simulink library "se_batching"  (Simulink 7.9)
settings: Solver=VariableStepDiscrete  SolverMode=SingleTasking  StartTime=0.0  StopTime=inf  RelTol=1e-3
libraries: simulink x7
settings Model: Creator=rrosson  LastModifiedBy=tsprock3

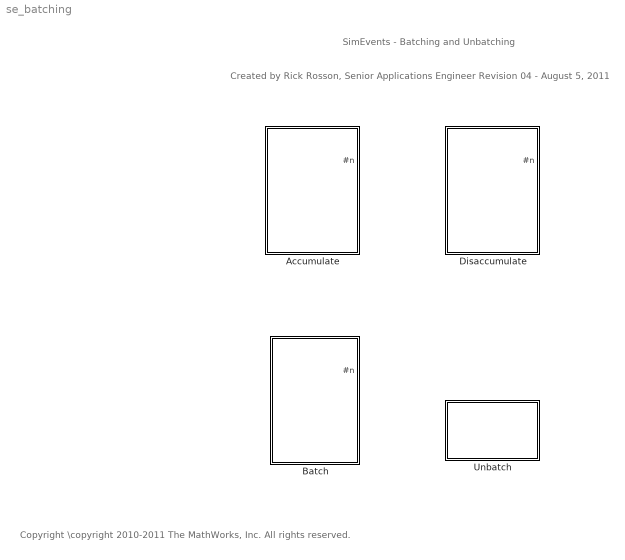
== system se_batching ==
  note: Copyright \copyright 2010-2011 The MathWorks, Inc. All rights reserved.
  note: SimEvents - Batching and Unbatching
  note: Created by Rick Rosson, Senior Applications Engineer
      | Revision 04 - August 5, 2011
  Accumulate : Subsystem  mask(Accumulate){Q=20}
      mask prompts: Q "Bach quantity (entities/batch), Q ="
      mask help:
      | Takes in entities and stores them until the number of entities stored reaches a specified number called the batch quantity.  The block then passes all of the stored entities to the output simultaneously.
      | The #n output signal provides the number of entities stored in the block at each time step.
      mask init:
      | if Q < 2
      |     error('Q must be greater than 1');
      | end
  Batch : Subsystem  mask(Batch){Q=20}
      mask prompts: Q "Bach quantity (entities/batch), Q ="
      mask help:
      | Takes in entities and stores them until the number of entities stored reaches a specified number called the batch quantity.  The block then generates a single entity, which represents a batch, and passes the batch entity to the output.
      | The #n output signal provides the number of entities stored in the block at each time step.
      mask init:
      | if Q < 2
      |     error('Q must be greater than 1');
      | end
  Disaccumulate : Subsystem  mask(Disaccumulaton){Qmax=inf, Nmax=inf, Tc=1}
      mask prompts: Qmax "Maxiumum batch size (entities per batch), Qmax"; Nmax "Maximum number of batches, Nmax ="; Tc "Cycle time, Tc ="
  Unbatch : Subsystem  mask(Unbatch){Q=20}
      mask prompts: Q "Batch quantity (entities/batch), Q ="
      mask help: Takes a single entity representing a batch and converts it into multiple entities. A parameter determines the batch quantity, which is the number of entities generated at the output for each entity arriving at the input.
      mask init:
      | if Q < 2
      |     error('Q must be greater than 1');
      | end

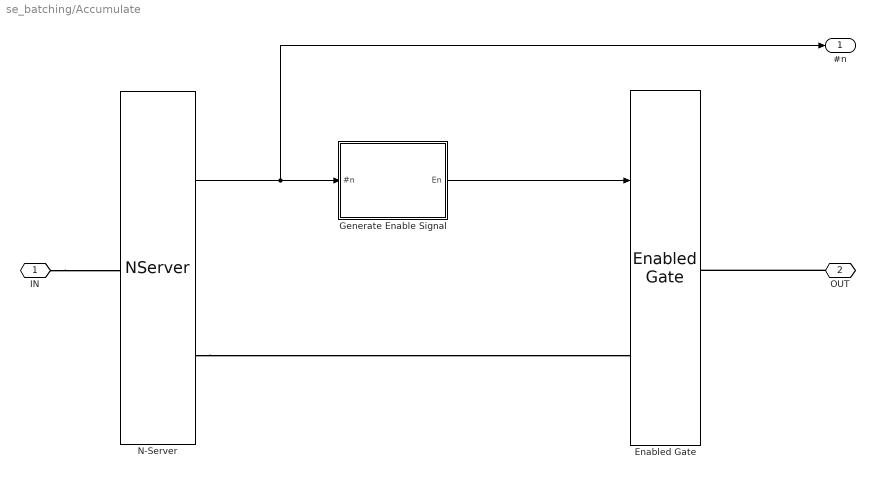
== system se_batching/Accumulate ==
  Enabled Gate : EnabledGate
  Generate Enable Signal : Subsystem
  N-Server : NServer  NumberOfServers=Q  ServiceTime=0  StatNumberInBlock=on
      settings: OutputPortMap=o1
  IN : PMIOPort  Port=1  Side=Left
  OUT : PMIOPort  Port=2  Side=Right
  #n : Outport
  wires:
  Generate Enable Signal/1(En) -> Enabled Gate/1
  N-Server/1 -> #n/1, Generate Enable Signal/1(#n)
  connections:
  OUT/RConn1 -- Enabled Gate/RConn1
  IN/RConn1 -- N-Server/LConn1
  N-Server/RConn1 -- Enabled Gate/LConn1

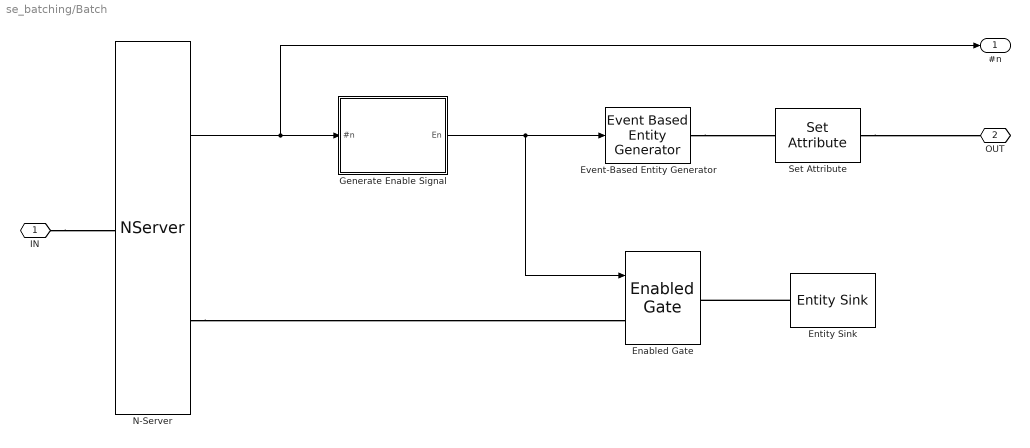
== system se_batching/Batch ==
  Enabled Gate : EnabledGate
  Entity Sink : EntitySink
  Event-Based Entity Generator : EventBasedEntityGenerator
  Generate Enable Signal : Subsystem
  N-Server : NServer  NumberOfServers=Q  ServiceTime=0  StatNumberInBlock=on
      settings: OutputPortMap=o1
  Set Attribute : SetAttribute  AttributeName=BatchQuantity  AttributeValue=Q  EvaluatedAttributeValue={Q}
  IN : PMIOPort  Port=1  Side=Left
  OUT : PMIOPort  Port=2  Side=Right
  #n : Outport
  wires:
  N-Server/1 -> Generate Enable Signal/1(#n), #n/1
  Generate Enable Signal/1(En) -> Enabled Gate/1, Event-Based Entity Generator/1
  connections:
  N-Server/RConn1 -- Enabled Gate/LConn1
  IN/RConn1 -- N-Server/LConn1
  Entity Sink/LConn1 -- Enabled Gate/RConn1
  Event-Based Entity Generator/RConn1 -- Set Attribute/LConn1
  Set Attribute/RConn1 -- OUT/RConn1

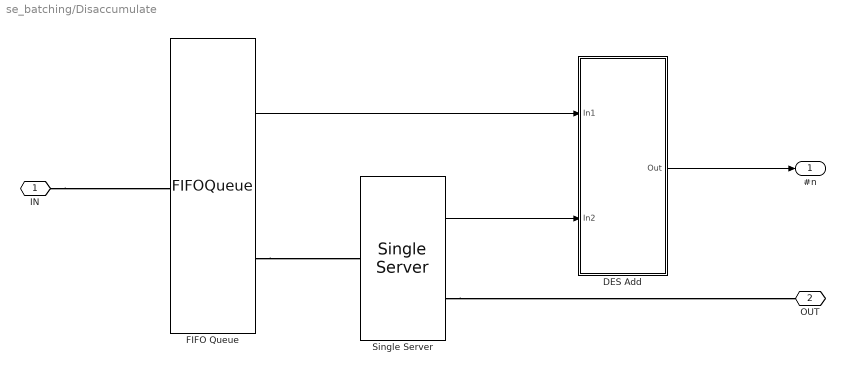
== system se_batching/Disaccumulate ==
  DES Add : Subsystem
  FIFO Queue : FIFOQueue  Capacity=Qmax*Nmax  StatNumberInBlock=on
      settings: OutputPortMap=o1
  Single Server : SingleServer  ServiceTime=Tc  StatNumberInBlock=on
      settings: OutputPortMap=o1
  IN : PMIOPort  Port=1  Side=Left
  OUT : PMIOPort  Port=2  Side=Right
  #n : Outport
  wires:
  Single Server/1 -> DES Add/2(In2)
  FIFO Queue/1 -> DES Add/1(In1)
  DES Add/1(Out) -> #n/1
  connections:
  Single Server/RConn1 -- OUT/RConn1
  IN/RConn1 -- FIFO Queue/LConn1
  FIFO Queue/RConn1 -- Single Server/LConn1

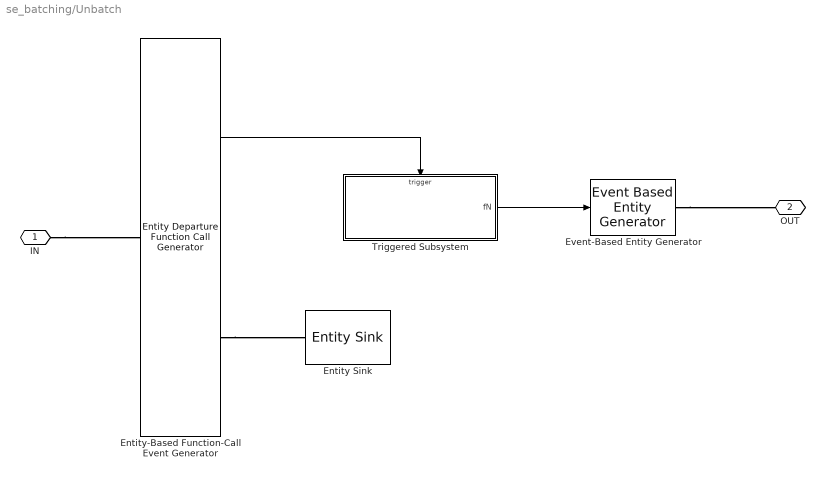
== system se_batching/Unbatch ==
  Entity Sink : EntitySink
  Entity-Based Function-Call Event Generator : EntityDepartureFunctionCallGenerator  TimingFunctionCallF2=After entity departure
  Event-Based Entity Generator : EventBasedEntityGenerator  GenerateEntitiesUpon=Function call from port fcn
  Triggered Subsystem : Subsystem  TreatAsAtomicUnit=on
  IN : PMIOPort  Port=1  Side=Left
  OUT : PMIOPort  Port=2  Side=Right
  wires:
  Entity-Based Function-Call Event Generator/1 -> Triggered Subsystem/Trigger
  Triggered Subsystem/1(fN) -> Event-Based Entity Generator/1
  connections:
  IN/RConn1 -- Entity-Based Function-Call Event Generator/LConn1
  Entity-Based Function-Call Event Generator/RConn1 -- Entity Sink/LConn1
  Event-Based Entity Generator/RConn1 -- OUT/RConn1

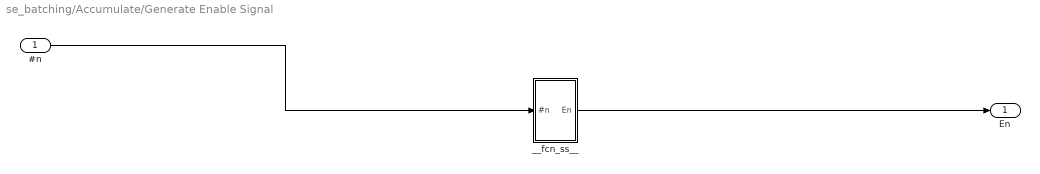
== system se_batching/Accumulate/Generate Enable Signal ==
  #n : Inport
  __fcn_ss__ : Subsystem  TreatAsAtomicUnit=on
  En : Outport
  wires:
  __fcn_ss__/1(En) -> En/1
  #n/1 -> __fcn_ss__/1(#n)

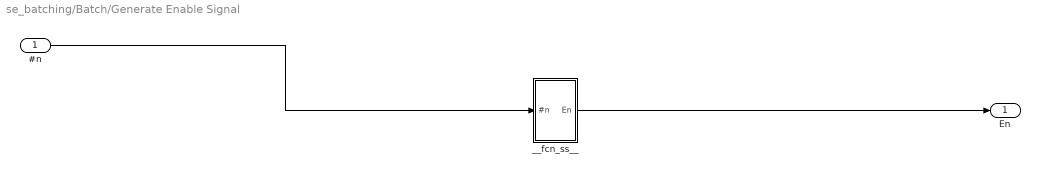
== system se_batching/Batch/Generate Enable Signal ==
  #n : Inport
  __fcn_ss__ : Subsystem  TreatAsAtomicUnit=on
  En : Outport
  wires:
  __fcn_ss__/1(En) -> En/1
  #n/1 -> __fcn_ss__/1(#n)

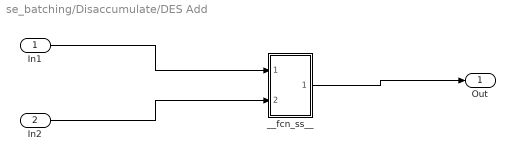
== system se_batching/Disaccumulate/DES Add ==
  In1 : Inport
  In2 : Inport  Port=2
  __fcn_ss__ : Subsystem  TreatAsAtomicUnit=on
  Out : Outport
  wires:
  __fcn_ss__/1(Out) -> Out/1
  In2/1 -> __fcn_ss__/2(In2)
  In1/1 -> __fcn_ss__/1(In1)

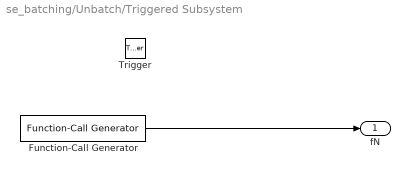
== system se_batching/Unbatch/Triggered Subsystem ==
  Trigger : TriggerPort  TriggerType=function-call
  Function-Call Generator : simulink/Ports & Subsystems/Function-Call Generator  sample_time=-1  numberOfIterations=Q
  fN : Outport
  wires:
  Function-Call Generator/1 -> fN/1

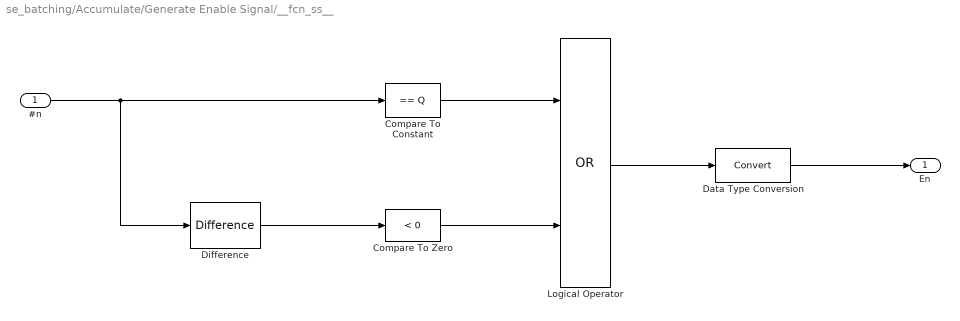
== system se_batching/Accumulate/Generate Enable Signal/__fcn_ss__ ==
  #n : Inport
  Compare To Constant : simulink/Logic and Bit Operations/Compare To Constant  relop===  const=Q  OutDataTypeStr=boolean
  Compare To Zero : simulink/Logic and Bit Operations/Compare To Zero  relop=<  OutDataTypeStr=boolean
  Data Type Conversion : DataTypeConversion
  Difference : simulink/Discrete/Difference  ICPrevInput=0.0  InputProcessing=Inherited  OutMin=[]  OutMax=[]  OutDataType=fixdt(1, 16)  OutScaling=2^-10  DoSatur=off
  Logical Operator : Logic  Operator=OR  AllPortsSameDT=off  OutDataTypeStr=boolean
  En : Outport
  wires:
  Compare To Zero/1 -> Logical Operator/2
  Difference/1 -> Compare To Zero/1
  Logical Operator/1 -> Data Type Conversion/1
  Compare To Constant/1 -> Logical Operator/1
  #n/1 -> Difference/1, Compare To Constant/1
  Data Type Conversion/1 -> En/1

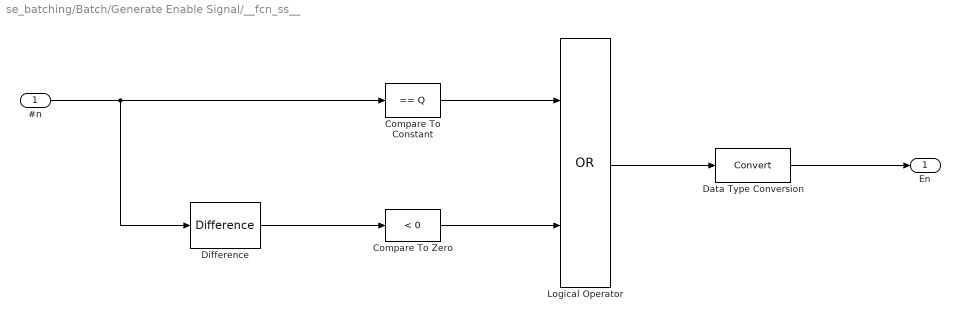
== system se_batching/Batch/Generate Enable Signal/__fcn_ss__ ==
  #n : Inport
  Compare To Constant : simulink/Logic and Bit Operations/Compare To Constant  relop===  const=Q  OutDataTypeStr=boolean
  Compare To Zero : simulink/Logic and Bit Operations/Compare To Zero  relop=<  OutDataTypeStr=boolean
  Data Type Conversion : DataTypeConversion
  Difference : simulink/Discrete/Difference  ICPrevInput=0.0  InputProcessing=Inherited  OutMin=[]  OutMax=[]  OutDataType=fixdt(1, 16)  OutScaling=2^-10  DoSatur=off
  Logical Operator : Logic  Operator=OR  AllPortsSameDT=off  OutDataTypeStr=boolean
  En : Outport
  wires:
  Data Type Conversion/1 -> En/1
  #n/1 -> Compare To Constant/1, Difference/1
  Compare To Constant/1 -> Logical Operator/1
  Logical Operator/1 -> Data Type Conversion/1
  Difference/1 -> Compare To Zero/1
  Compare To Zero/1 -> Logical Operator/2

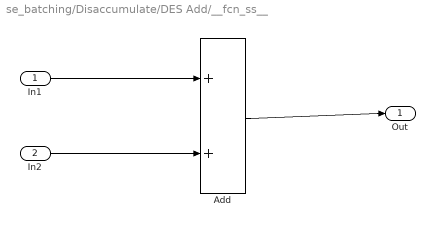
== system se_batching/Disaccumulate/DES Add/__fcn_ss__ ==
  In1 : Inport
  In2 : Inport  Port=2
  Add : Sum
  Out : Outport
  wires:
  Add/1 -> Out/1
  In1/1 -> Add/1
  In2/1 -> Add/2
